simulink model "ModelN_PID"  (R2022b)
settings: Solver=VariableStepAuto  StartTime=0.0  StopTime=50  RelTol=1e-3
values from neighbouring files (symbols this model uses):
  Ix = 7.5e-3    (= 0.0075)    [values_1.m]
  Iy = Ix    (= 0.0075)    [values_1.m]
  Iz = 1.3e-2    (= 0.013)    [values_1.m]
  l = 1    [values_1.m]
undefined symbols (not defined in the file or in its folder): sigbuilder_block
libraries: slpidlib x3, simulink x1
settings Model: Creator=kumar  LastModifiedBy=Niku

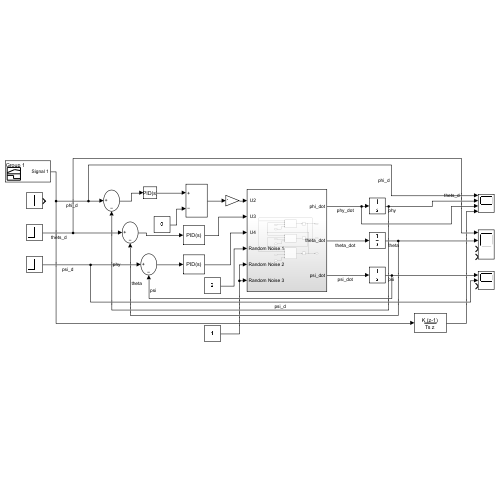
[thumbnail: Simulink's stored preview of the top-level diagram]
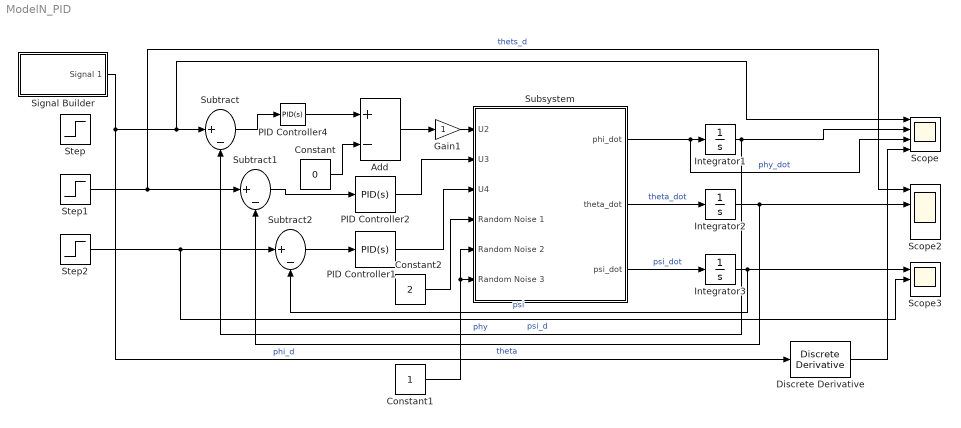
== system ModelN_PID ==
  Add : Sum  Inputs=+-
  Constant : Constant  Value=0
  Constant1 : Constant
  Constant2 : Constant  Value=2
  Discrete Derivative : simulink/Discrete/Discrete Derivative  gainval=1.0  ICPrevScaledInput=0.0  OutMin=[]  OutMax=[]  OutDataType=fixdt(1, 16)  OutScaling=2^-10  DoSatur=off
  Gain1 : Gain
  Integrator1 : Integrator
  Integrator2 : Integrator
  Integrator3 : Integrator
  PID Controller1 : slpidlib/PID Controller  Controller=PID  Form=Parallel  TimeDomain=Continuous-time  UseExternalTs=off  SampleTime=-1  IntegratorMethod=Forward Euler  FilterMethod=Forward Euler  ControllerParametersSource=internal  P=-0.00241383042252482  I=-0.000113002936035472  UseKiTs=off  D=-0.0126609727607765  N=5.45397025421619  UseFilter=on  TunerSelectOption=Transfer Function Based (PID Tuner App)  InitialConditionSource=internal  InitialConditionForIntegrator=0  InitialConditionForFilter=0  DifferentiatorICPrevScaledInput=0  ExternalReset=none  TrackingMode=off  Kt=1  LimitOutput=off  SatLimitsSource=internal  UpperSaturationLimit=inf  LowerSaturationLimit=-inf  LinearizeAsGain=on  AntiWindupMode=none  Kb=1  LimitIntegrator=off  UpperIntegratorSaturationLimit=inf  LowerIntegratorSaturationLimit=-inf  POutMin=[]  POutMax=[]  IOutMin=[]  IOutMax=[]  DOutMin=[]  DOutMax=[]  NOutMin=[]  NOutMax=[]  SumOutMin=[]  SumOutMax=[]  SaturationOutMin=[]  SaturationOutMax=[]  PParamMin=[]  PParamMax=[]  IParamMin=[]  IParamMax=[]  DParamMin=[]  DParamMax=[]  NParamMin=[]  NParamMax=[]  KbParamMin=[]  KbParamMax=[]  KtParamMin=[]  KtParamMax=[]  KbOutMin=[]  KbOutMax=[]  KtOutMin=[]  KtOutMax=[]  IntegratorOutMin=[]  IntegratorOutMax=[]  FilterOutMin=[]  FilterOutMax=[]  SumI1OutMin=[]  SumI1OutMax=[]  SumI2OutMin=[]  SumI2OutMax=[]  SumI3OutMin=[]  SumI3OutMax=[]  SumI4OutMin=[]  SumI4OutMax=[]  SumDOutMin=[]  SumDOutMax=[]  DifferentiatorOutMin=[]  DifferentiatorOutMax=[]  FilterDiffOutCoefMin=[]  FilterDiffOutCoefMax=[]  ReciprocalOutMin=[]  ReciprocalOutMax=[]  SumDenOutMin=[]  SumDenOutMax=[]  SumNumOutMin=[]  SumNumOutMax=[]  DivideOutMin=[]  DivideOutMax=[]  UdiffTsProdOutMin=[]  UdiffTsProdOutMax=[]  NTsProdOutMin=[]  NTsProdOutMax=[]  UintegralTsProdOutMin=[]  UintegralTsProdOutMax=[]  UngainTsProdOutMin=[]  UngainTsProdOutMax=[]  ClampingZeroOutDataTypeStr=Inherit: Inherit via back propagation  ClampingZeroOutMin=[]  ClampingZeroOutMax=[]  FilterDenConstantOutDataTypeStr=Inherit: Inherit via back propagation  FilterDenConstantOutMin=[]  FilterDenConstantOutMax=[]  PCopyOutDataTypeStr=Inherit: Inherit via back propagation  PCopyOutMin=[]  PCopyOutMax=[]  NCopyOutDataTypeStr=Inherit: Inherit via back propagation  NCopyOutMin=[]  NCopyOutMax=[]  IntegratorContinuousStateAttributes=''  IntegratorStateMustResolveToSignalObject=off  IntegratorRTWStateStorageClass=Auto  FilterContinuousStateAttributes=''  FilterStateMustResolveToSignalObject=off  FilterRTWStateStorageClass=Auto  ParallelPVariant=InternalParameters  IdealPVariant=Disabled  IVariant=InternalParameters  DVariant=InternalParameters  IntegratorVariant=Continuous  SatVariant=Disabled  AWVariant=Passthrough  PCopyVariant=Disabled  TRVariant=Disabled  FdbkBlocksVariant=Forward  IdealPFdbkVariant=Disabled  SatFdbkVariant=Disabled  DerivativeFilterVariant=ContFilter  NVariant=InternalParameters  NCopyVariant=Disabled  FilterICVariant=InternalICsFilter  IntegratorICVariant=InternalICs  ExternalResetVariant=Disabled  TRSumVariant=Passthrough  SumFdbkVariant=Disabled  SumVariant=Sum_PID  TsampFilterVariant=InternalTs  TsampNgainVariant=Passthrough  TsampIntegralVariant=Passthrough  ExternalSaturationOutDataTypeStr=Inherit: Same as second input
  PID Controller2 : slpidlib/PID Controller  Controller=PID  Form=Parallel  TimeDomain=Continuous-time  UseExternalTs=off  SampleTime=-1  IntegratorMethod=Forward Euler  FilterMethod=Forward Euler  ControllerParametersSource=internal  P=-0.0605475858492847  I=-0.00896354498725105  UseKiTs=off  D=-0.100428540093823  N=17.2469682941307  UseFilter=on  TunerSelectOption=Transfer Function Based (PID Tuner App)  InitialConditionSource=internal  InitialConditionForIntegrator=0  InitialConditionForFilter=0  DifferentiatorICPrevScaledInput=0  ExternalReset=none  TrackingMode=off  Kt=1  LimitOutput=off  SatLimitsSource=internal  UpperSaturationLimit=inf  LowerSaturationLimit=-inf  LinearizeAsGain=on  AntiWindupMode=none  Kb=1  LimitIntegrator=off  UpperIntegratorSaturationLimit=inf  LowerIntegratorSaturationLimit=-inf  POutMin=[]  POutMax=[]  IOutMin=[]  IOutMax=[]  DOutMin=[]  DOutMax=[]  NOutMin=[]  NOutMax=[]  SumOutMin=[]  SumOutMax=[]  SaturationOutMin=[]  SaturationOutMax=[]  PParamMin=[]  PParamMax=[]  IParamMin=[]  IParamMax=[]  DParamMin=[]  DParamMax=[]  NParamMin=[]  NParamMax=[]  KbParamMin=[]  KbParamMax=[]  KtParamMin=[]  KtParamMax=[]  KbOutMin=[]  KbOutMax=[]  KtOutMin=[]  KtOutMax=[]  IntegratorOutMin=[]  IntegratorOutMax=[]  FilterOutMin=[]  FilterOutMax=[]  SumI1OutMin=[]  SumI1OutMax=[]  SumI2OutMin=[]  SumI2OutMax=[]  SumI3OutMin=[]  SumI3OutMax=[]  SumI4OutMin=[]  SumI4OutMax=[]  SumDOutMin=[]  SumDOutMax=[]  DifferentiatorOutMin=[]  DifferentiatorOutMax=[]  FilterDiffOutCoefMin=[]  FilterDiffOutCoefMax=[]  ReciprocalOutMin=[]  ReciprocalOutMax=[]  SumDenOutMin=[]  SumDenOutMax=[]  SumNumOutMin=[]  SumNumOutMax=[]  DivideOutMin=[]  DivideOutMax=[]  UdiffTsProdOutMin=[]  UdiffTsProdOutMax=[]  NTsProdOutMin=[]  NTsProdOutMax=[]  UintegralTsProdOutMin=[]  UintegralTsProdOutMax=[]  UngainTsProdOutMin=[]  UngainTsProdOutMax=[]  ClampingZeroOutDataTypeStr=Inherit: Inherit via back propagation  ClampingZeroOutMin=[]  ClampingZeroOutMax=[]  FilterDenConstantOutDataTypeStr=Inherit: Inherit via back propagation  FilterDenConstantOutMin=[]  FilterDenConstantOutMax=[]  PCopyOutDataTypeStr=Inherit: Inherit via back propagation  PCopyOutMin=[]  PCopyOutMax=[]  NCopyOutDataTypeStr=Inherit: Inherit via back propagation  NCopyOutMin=[]  NCopyOutMax=[]  IntegratorContinuousStateAttributes=''  IntegratorStateMustResolveToSignalObject=off  IntegratorRTWStateStorageClass=Auto  FilterContinuousStateAttributes=''  FilterStateMustResolveToSignalObject=off  FilterRTWStateStorageClass=Auto  ParallelPVariant=InternalParameters  IdealPVariant=Disabled  IVariant=InternalParameters  DVariant=InternalParameters  IntegratorVariant=Continuous  SatVariant=Disabled  AWVariant=Passthrough  PCopyVariant=Disabled  TRVariant=Disabled  FdbkBlocksVariant=Forward  IdealPFdbkVariant=Disabled  SatFdbkVariant=Disabled  DerivativeFilterVariant=ContFilter  NVariant=InternalParameters  NCopyVariant=Disabled  FilterICVariant=InternalICsFilter  IntegratorICVariant=InternalICs  ExternalResetVariant=Disabled  TRSumVariant=Passthrough  SumFdbkVariant=Disabled  SumVariant=Sum_PID  TsampFilterVariant=InternalTs  TsampNgainVariant=Passthrough  TsampIntegralVariant=Passthrough  ExternalSaturationOutDataTypeStr=Inherit: Same as second input
  PID Controller4 : slpidlib/PID Controller  Controller=PID  Form=Parallel  TimeDomain=Continuous-time  UseExternalTs=off  SampleTime=-1  IntegratorMethod=Forward Euler  FilterMethod=Forward Euler  ControllerParametersSource=internal  P=0.315299517595255  I=0.111408292309888  UseKiTs=off  D=0.219927172885629  N=72.5711011508283  UseFilter=on  TunerSelectOption=Transfer Function Based (PID Tuner App)  InitialConditionSource=internal  InitialConditionForIntegrator=0  InitialConditionForFilter=0  DifferentiatorICPrevScaledInput=0  ExternalReset=none  TrackingMode=off  Kt=1  LimitOutput=off  SatLimitsSource=internal  UpperSaturationLimit=inf  LowerSaturationLimit=-inf  LinearizeAsGain=on  AntiWindupMode=none  Kb=1  LimitIntegrator=off  UpperIntegratorSaturationLimit=inf  LowerIntegratorSaturationLimit=-inf  POutMin=[]  POutMax=[]  IOutMin=[]  IOutMax=[]  DOutMin=[]  DOutMax=[]  NOutMin=[]  NOutMax=[]  SumOutMin=[]  SumOutMax=[]  SaturationOutMin=[]  SaturationOutMax=[]  PParamMin=[]  PParamMax=[]  IParamMin=[]  IParamMax=[]  DParamMin=[]  DParamMax=[]  NParamMin=[]  NParamMax=[]  KbParamMin=[]  KbParamMax=[]  KtParamMin=[]  KtParamMax=[]  KbOutMin=[]  KbOutMax=[]  KtOutMin=[]  KtOutMax=[]  IntegratorOutMin=[]  IntegratorOutMax=[]  FilterOutMin=[]  FilterOutMax=[]  SumI1OutMin=[]  SumI1OutMax=[]  SumI2OutMin=[]  SumI2OutMax=[]  SumI3OutMin=[]  SumI3OutMax=[]  SumI4OutMin=[]  SumI4OutMax=[]  SumDOutMin=[]  SumDOutMax=[]  DifferentiatorOutMin=[]  DifferentiatorOutMax=[]  FilterDiffOutCoefMin=[]  FilterDiffOutCoefMax=[]  ReciprocalOutMin=[]  ReciprocalOutMax=[]  SumDenOutMin=[]  SumDenOutMax=[]  SumNumOutMin=[]  SumNumOutMax=[]  DivideOutMin=[]  DivideOutMax=[]  UdiffTsProdOutMin=[]  UdiffTsProdOutMax=[]  NTsProdOutMin=[]  NTsProdOutMax=[]  UintegralTsProdOutMin=[]  UintegralTsProdOutMax=[]  UngainTsProdOutMin=[]  UngainTsProdOutMax=[]  ClampingZeroOutDataTypeStr=Inherit: Inherit via back propagation  ClampingZeroOutMin=[]  ClampingZeroOutMax=[]  FilterDenConstantOutDataTypeStr=Inherit: Inherit via back propagation  FilterDenConstantOutMin=[]  FilterDenConstantOutMax=[]  PCopyOutDataTypeStr=Inherit: Inherit via back propagation  PCopyOutMin=[]  PCopyOutMax=[]  NCopyOutDataTypeStr=Inherit: Inherit via back propagation  NCopyOutMin=[]  NCopyOutMax=[]  IntegratorContinuousStateAttributes=''  IntegratorStateMustResolveToSignalObject=off  IntegratorRTWStateStorageClass=Auto  FilterContinuousStateAttributes=''  FilterStateMustResolveToSignalObject=off  FilterRTWStateStorageClass=Auto  ParallelPVariant=InternalParameters  IdealPVariant=Disabled  IVariant=InternalParameters  DVariant=InternalParameters  IntegratorVariant=Continuous  SatVariant=Disabled  AWVariant=Passthrough  PCopyVariant=Disabled  TRVariant=Disabled  FdbkBlocksVariant=Forward  IdealPFdbkVariant=Disabled  SatFdbkVariant=Disabled  DerivativeFilterVariant=ContFilter  NVariant=InternalParameters  NCopyVariant=Disabled  FilterICVariant=InternalICsFilter  IntegratorICVariant=InternalICs  ExternalResetVariant=Disabled  TRSumVariant=Passthrough  SumFdbkVariant=Disabled  SumVariant=Sum_PID  TsampFilterVariant=InternalTs  TsampNgainVariant=Passthrough  TsampIntegralVariant=Passthrough  ExternalSaturationOutDataTypeStr=Inherit: Same as second input
  Scope : Scope  NumInputPorts=4
  Scope2 : Scope  NumInputPorts=4
  Scope3 : Scope  NumInputPorts=3
  Signal Builder : Subsystem  Tag=STV Subsys  LoadFcn=sigbuilder_block('load');  StartFcn=sigbuilder_block('start');  StopFcn=sigbuilder_block('stop');  ClipboardFcn=sigbuilder_block('clipboard');  mask(Sigbuilder block){tuvar=[0:10]}
      mask help: Simulink:masks:SigbuilderBlock_MD
      mask init:
      | if ~strcmp(get_param(bdroot(gcbh),'SimulationStatus'),'stopped') tuvar = sigbuilder_block('maskInit'); end
      settings: CopyFcn=sigbuilder_block('copy');  DeleteFcn=sigbuilder_block('delete');  ModelCloseFcn=sigbuilder_block('modelClose');  PreSaveFcn=sigbuilder_block('preSave');  PauseFcn=sigbuilder_block('pause');  ContinueFcn=sigbuilder_block('continue');  NameChangeFcn=sigbuilder_block('namechange');  OpenFcn=sigbuilder_block('open',[0 36 1024.5 482.25 ]);  CloseFcn=sigbuilder_block('close');
      mask Display: plot(0, 0, 100, 100,[2, 2, 32, 32, 2], [68, 8, 8, 68, 68],[32, 2], [38, 38], [32, 19, 2],[53, 60, 44], [32, 17, 17, 2],[16, 16, 31, 31]);txt = getActiveGroup(gcbh);text(2, 100, txt,'verticalAlignment', 'top');
  Step : Step  SampleTime=0
  Step1 : Step  After=2  SampleTime=0
  Step2 : Step  After=3  SampleTime=0
  Subsystem : Subsystem
  Subtract : Sum  Inputs=|+-
  Subtract1 : Sum  Inputs=|+-
  Subtract2 : Sum  Inputs=|+-
  wires:
  Subsystem/1(phi_dot) -> Scope/3, Integrator1/1  "phy_dot"
  Subsystem/2(theta_dot) -> Integrator2/1  "theta_dot"
  Subsystem/3(psi_dot) -> Integrator3/1  "psi_dot"
  Integrator1/1 -> Scope/2, Subtract/2  "phy"
  Integrator2/1 -> Subtract1/2, Scope2/2  "theta"
  Integrator3/1 -> Scope3/1, Subtract2/2  "psi"
  Constant1/1 -> Subsystem/5(Random Noise 2), Subsystem/6(Random Noise 3)
  Constant2/1 -> Subsystem/4(Random Noise 1)
  Signal Builder/1(Signal 1) -> Discrete Derivative/1, Subtract/1, Scope/1  "phi_d"
  Step1/1 -> Subtract1/1, Scope2/1  "thets_d"
  PID Controller1/1 -> Subsystem/3(" U4")
  Subtract2/1 -> PID Controller1/1
  Step2/1 -> Scope3/2, Subtract2/1  "psi_d"
  Add/1 -> Gain1/1
  Gain1/1 -> Subsystem/1(" U2")
  Subtract1/1 -> PID Controller2/1
  PID Controller2/1 -> Subsystem/2(" U3")
  PID Controller4/1 -> Add/1
  Subtract/1 -> PID Controller4/1
  Constant/1 -> Add/2
  Discrete Derivative/1 -> Scope/4

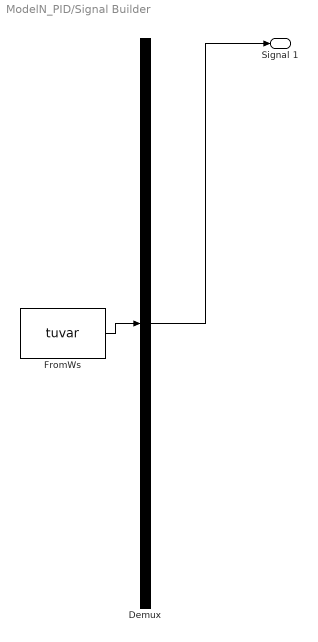
== system ModelN_PID/Signal Builder ==
  Demux : Demux  Tag=STV Demux  Outputs=1
      settings: DisplayOption=none
  FromWs : FromWorkspace  Tag=STV FromWs  VariableName=tuvar
      SigBuilderData=|
      | common.afterFinalStr = 'Extrapolate'
      | common.sampleTime = 0
      | dataSet.timeRange = [0 50]
      | dataSet.name = 'Group 1'
      | sbobj.Groups.Name = 'Group 1'
      | sbobj.Groups.Signals.Name = 'Signal 1'
      | sbobj.Groups.Signals.XData = [0 4 4 6 25 50]
      | sbobj.Groups.Signals.YData = [0 0 1 1 0 0]
      | sbobj.Groups.TimeRange = [0 50]
  Signal 1 : Outport  Tag=STV Outport
  wires:
  Demux/1 -> Signal 1/1
  FromWs/1 -> Demux/1

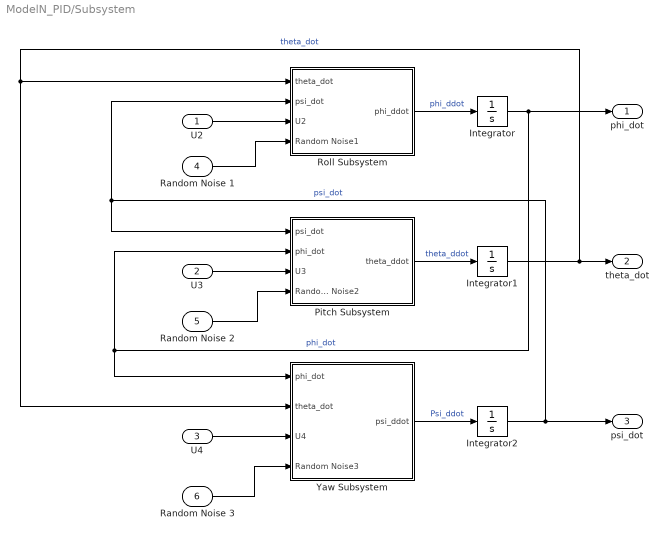
== system ModelN_PID/Subsystem ==
  " U2" : Inport
  " U3" : Inport  Port=2
  " U4" : Inport  Port=3
  Random Noise 1 : Inport  Port=4
  Random Noise 2 : Inport  Port=5
  Random Noise 3 : Inport  Port=6
  Integrator : Integrator
  Integrator1 : Integrator
  Integrator2 : Integrator
  Pitch Subsystem : Subsystem
  Roll Subsystem : Subsystem
  Yaw Subsystem : Subsystem
  phi_dot : Outport
  theta_dot : Outport  Port=2
  psi_dot : Outport  Port=3
  wires:
  " U2"/1 -> Roll Subsystem/3(" U2")
  Random Noise 1/1 -> Roll Subsystem/4(Random Noise1)
  Yaw Subsystem/1(psi_ddot) -> Integrator2/1  "Psi_ddot"
  " U3"/1 -> Pitch Subsystem/3(" U3")
  Random Noise 2/1 -> Pitch Subsystem/4(Random Noise2)
  " U4"/1 -> Yaw Subsystem/3(" U4")
  Random Noise 3/1 -> Yaw Subsystem/4(Random Noise3)
  Roll Subsystem/1(phi_ddot) -> Integrator/1  "phi_ddot"
  Pitch Subsystem/1(theta_ddot) -> Integrator1/1  "theta_ddot"
  Integrator/1 -> Yaw Subsystem/1(phi_dot), Pitch Subsystem/2(phi_dot), phi_dot/1  "phi_dot"
  Integrator1/1 -> theta_dot/1, Yaw Subsystem/2(theta_dot), Roll Subsystem/1(theta_dot)  "theta_dot"
  Integrator2/1 -> Pitch Subsystem/1(psi_dot), Roll Subsystem/2(psi_dot), psi_dot/1  "psi_dot"

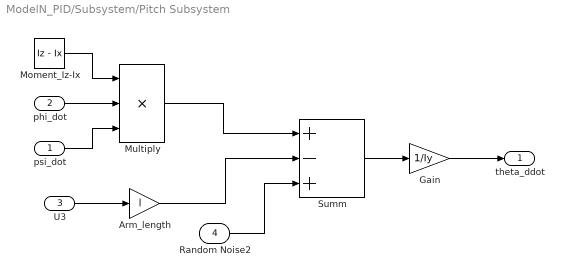
== system ModelN_PID/Subsystem/Pitch Subsystem ==
  psi_dot : Inport
  phi_dot : Inport  Port=2
  " U3" : Inport  Port=3
  Random Noise2 : Inport  Port=4
  Arm_length : Gain  Gain=l
  Gain : Gain  Gain=1/Iy
  Moment_Iz-Ix : Constant  Value=Iz - Ix
  Multiply : Product  Inputs=3
  Summ : Sum  Inputs=+-+
  theta_ddot : Outport
  wires:
  Gain/1 -> theta_ddot/1
  Moment_Iz-Ix/1 -> Multiply/1
  " U3"/1 -> Arm_length/1
  psi_dot/1 -> Multiply/3
  phi_dot/1 -> Multiply/2
  Multiply/1 -> Summ/1
  Arm_length/1 -> Summ/2
  Summ/1 -> Gain/1
  Random Noise2/1 -> Summ/3

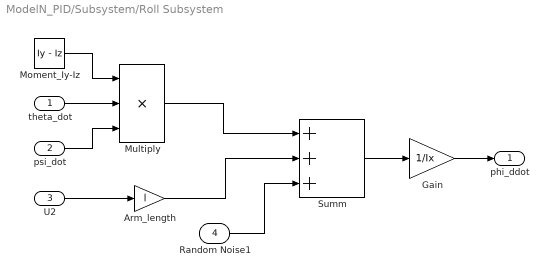
== system ModelN_PID/Subsystem/Roll Subsystem ==
  theta_dot : Inport
  psi_dot : Inport  Port=2
  " U2" : Inport  Port=3
  Random Noise1 : Inport  Port=4
  Arm_length : Gain  Gain=l
  Gain : Gain  Gain=1/Ix
  Moment_Iy-Iz : Constant  Value=Iy - Iz
  Multiply : Product  Inputs=3
  Summ : Sum  Inputs=+++
  phi_ddot : Outport
  wires:
  Summ/1 -> Gain/1
  Random Noise1/1 -> Summ/3
  " U2"/1 -> Arm_length/1
  Multiply/1 -> Summ/1
  psi_dot/1 -> Multiply/3
  Gain/1 -> phi_ddot/1
  Moment_Iy-Iz/1 -> Multiply/1
  theta_dot/1 -> Multiply/2
  Arm_length/1 -> Summ/2

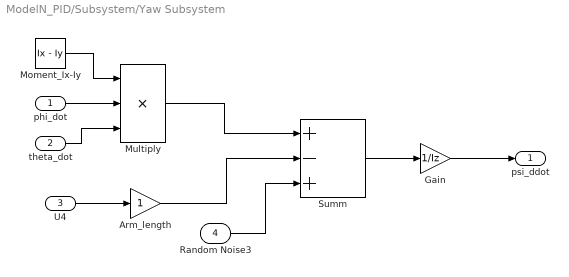
== system ModelN_PID/Subsystem/Yaw Subsystem ==
  phi_dot : Inport
  theta_dot : Inport  Port=2
  " U4" : Inport  Port=3
  Random Noise3 : Inport  Port=4
  Arm_length : Gain
  Gain : Gain  Gain=1/Iz
  Moment_Ix-Iy : Constant  Value=Ix - Iy
  Multiply : Product  Inputs=3
  Summ : Sum  Inputs=+-+
  psi_ddot : Outport
  wires:
  Summ/1 -> Gain/1
  " U4"/1 -> Arm_length/1
  Multiply/1 -> Summ/1
  Gain/1 -> psi_ddot/1
  Arm_length/1 -> Summ/2
  phi_dot/1 -> Multiply/2
  theta_dot/1 -> Multiply/3
  Random Noise3/1 -> Summ/3
  Moment_Ix-Iy/1 -> Multiply/1
